simulink model "cc_architecture_model"  (R2024a)
settings: Solver=VariableStepAuto  StartTime=0.0  StopTime=10.0  RelTol=1e-3
settings Model: Creator=nevil  LastModifiedBy=nevil

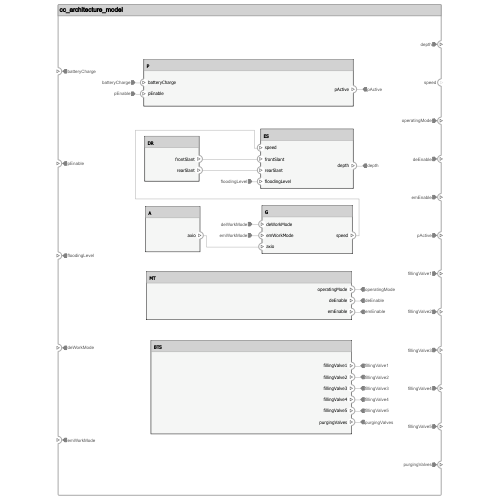
[thumbnail: Simulink's stored preview of the top-level diagram]
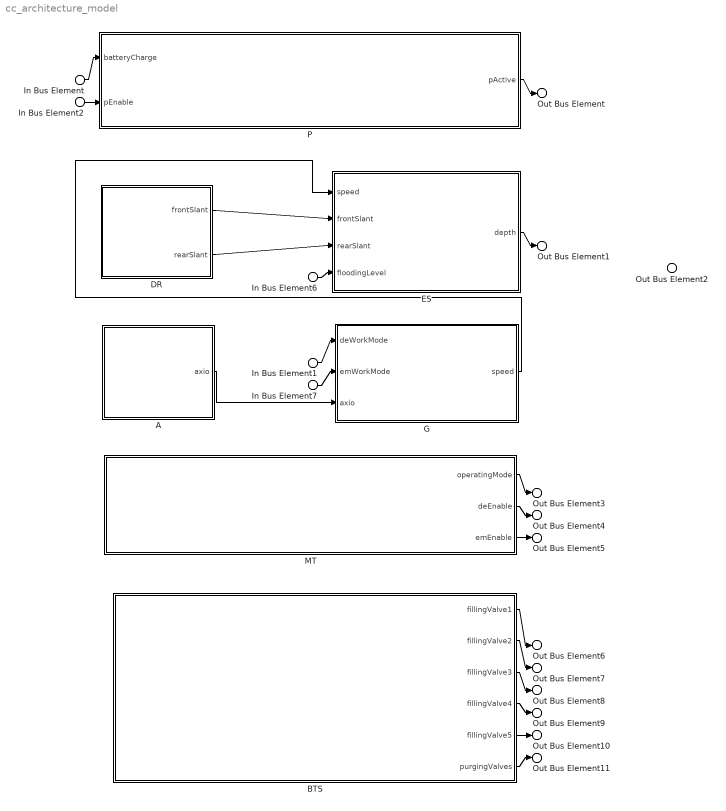
== system cc_architecture_model ==
  In Bus Element : Inport  PortName=batteryCharge
  In Bus Element2 : Inport  Port=2  PortName=pEnable
  In Bus Element6 : Inport  Port=3  PortName=floodingLevel
  In Bus Element1 : Inport  Port=4  PortName=deWorkMode
  In Bus Element7 : Inport  Port=5  PortName=emWorkMode
  A : Subsystem
      settings: PortSchema="{\"entries\":[{\"content\":{\"headerSize\":26,\"margin\":15,\"minimumSpacing\":25,\"sides\":[{\"content\":{},\"type\":\"ConnectorPlacement.EquallySpacedRectSide\",\"uuid\":\"55c3a500-c9db-403b-90f2-8c12a75bb2a5\"},{\"content\":{\"connectorIds\":[\"Out1\"],\"side\":\"RIGHT\"},\"type\":\"ConnectorPlacement.EquallySpacedRectSide\",\"uuid\":\"33fbbcf8-5fdb-46c8-86f1-27d61e7d7260\"},{\"content\":{\"side\":\"TOP\"},\"type\":\"ConnectorPlacement.EquallySpacedRectSide\",\"uuid\":\"56e8613f-dab0-46ca-a6c8-0c9dbbf33330\"}]},\"type\":\"ConnectorPlacement.EquallySpacedConnector\",\"uuid\":\"0944f535-9dc7-49a2-b8a9-c4d14048f3f3\"}],\"packageUris\":[\"http://schema.mathworks.com/mf0/Connector/R2020b\"],\"version\":\"1.0\"}"
  BTS : Subsystem
      settings: PortSchema="{\"entries\":[{\"content\":{\"headerSize\":26,\"margin\":15,\"minimumSpacing\":25,\"sides\":[{\"content\":{},\"type\":\"ConnectorPlacement.EquallySpacedRectSide\",\"uuid\":\"55c3a500-c9db-403b-90f2-8c12a75bb2a5\"},{\"content\":{\"connectorIds\":[\"Out1\",\"Out4\",\"Out3\",\"Out5\",\"Out2\",\"Out6\"],\"side\":\"RIGHT\"},\"type\":\"ConnectorPlacement.EquallySpacedRectSide\",\"uuid\":\"33fbbcf8-5fdb-46c8-86f1-27d61e7d7260\"},{\"content\":{\"side\":\"TOP\"},\"type\":\"ConnectorPlacement.EquallySpacedRectSide\",\"uuid\":\"56e8613f-dab0-46ca-a6c8-0c9dbbf33330\"}]},\"type\":\"ConnectorPlacement.EquallySpacedConnector\",\"uuid\":\"0944f535-9dc7-49a2-b8a9-c4d14048f3f3\"}],\"packageUris\":[\"http://schema.mathworks.com/mf0/Connector/R2020b\"],\"version\":\"1.0\"}"
  DR : Subsystem
      settings: PortSchema="{\"entries\":[{\"content\":{\"headerSize\":26,\"margin\":15,\"minimumSpacing\":25,\"sides\":[{\"content\":{},\"type\":\"ConnectorPlacement.EquallySpacedRectSide\",\"uuid\":\"55c3a500-c9db-403b-90f2-8c12a75bb2a5\"},{\"content\":{\"connectorIds\":[\"Out1\",\"Out2\"],\"side\":\"RIGHT\"},\"type\":\"ConnectorPlacement.EquallySpacedRectSide\",\"uuid\":\"33fbbcf8-5fdb-46c8-86f1-27d61e7d7260\"},{\"content\":{\"side\":\"TOP\"},\"type\":\"ConnectorPlacement.EquallySpacedRectSide\",\"uuid\":\"56e8613f-dab0-46ca-a6c8-0c9dbbf33330\"}]},\"type\":\"ConnectorPlacement.EquallySpacedConnector\",\"uuid\":\"0944f535-9dc7-49a2-b8a9-c4d14048f3f3\"}],\"packageUris\":[\"http://schema.mathworks.com/mf0/Connector/R2020b\"],\"version\":\"1.0\"}"
  ES : Subsystem
      settings: PortSchema="{\"entries\":[{\"content\":{\"headerSize\":26,\"margin\":15,\"minimumSpacing\":25,\"sides\":[{\"content\":{\"connectorIds\":[\"In1\",\"In2\",\"In3\",\"In4\"]},\"type\":\"ConnectorPlacement.EquallySpacedRectSide\",\"uuid\":\"fa34cfae-5758-447a-bbf8-61d94a7fad4b\"},{\"content\":{\"connectorIds\":[\"Out1\"],\"side\":\"RIGHT\"},\"type\":\"ConnectorPlacement.EquallySpacedRectSide\",\"uuid\":\"7d4a19cd-78f9-4f0a-b8b3-33613e9a47ea\"},{\"content\":{\"side\":\"TOP\"},\"type\":\"ConnectorPlacement.EquallySpacedRectSide\",\"uuid\":\"1bc8434e-3997-4d7a-991c-af8f97ade000\"}]},\"type\":\"ConnectorPlacement.EquallySpacedConnector\",\"uuid\":\"92e50b70-b613-4fba-b77c-cfd755548065\"}],\"packageUris\":[\"http://schema.mathworks.com/mf0/Connector/R2020b\"],\"version\":\"1.0\"}"
  G : Subsystem
      settings: PortSchema="{\"entries\":[{\"content\":{\"headerSize\":26,\"margin\":15,\"minimumSpacing\":25,\"sides\":[{\"content\":{\"connectorIds\":[\"In1\",\"In2\",\"In3\"]},\"type\":\"ConnectorPlacement.EquallySpacedRectSide\",\"uuid\":\"55c3a500-c9db-403b-90f2-8c12a75bb2a5\"},{\"content\":{\"connectorIds\":[\"Out1\"],\"side\":\"RIGHT\"},\"type\":\"ConnectorPlacement.EquallySpacedRectSide\",\"uuid\":\"33fbbcf8-5fdb-46c8-86f1-27d61e7d7260\"},{\"content\":{\"side\":\"TOP\"},\"type\":\"ConnectorPlacement.EquallySpacedRectSide\",\"uuid\":\"56e8613f-dab0-46ca-a6c8-0c9dbbf33330\"}]},\"type\":\"ConnectorPlacement.EquallySpacedConnector\",\"uuid\":\"0944f535-9dc7-49a2-b8a9-c4d14048f3f3\"}],\"packageUris\":[\"http://schema.mathworks.com/mf0/Connector/R2020b\"],\"version\":\"1.0\"}"
  MT : Subsystem
      settings: PortSchema="{\"entries\":[{\"content\":{\"headerSize\":26,\"margin\":15,\"minimumSpacing\":25,\"sides\":[{\"content\":{},\"type\":\"ConnectorPlacement.EquallySpacedRectSide\",\"uuid\":\"55c3a500-c9db-403b-90f2-8c12a75bb2a5\"},{\"content\":{\"connectorIds\":[\"Out1\",\"Out2\",\"Out3\"],\"side\":\"RIGHT\"},\"type\":\"ConnectorPlacement.EquallySpacedRectSide\",\"uuid\":\"33fbbcf8-5fdb-46c8-86f1-27d61e7d7260\"},{\"content\":{\"side\":\"TOP\"},\"type\":\"ConnectorPlacement.EquallySpacedRectSide\",\"uuid\":\"56e8613f-dab0-46ca-a6c8-0c9dbbf33330\"}]},\"type\":\"ConnectorPlacement.EquallySpacedConnector\",\"uuid\":\"0944f535-9dc7-49a2-b8a9-c4d14048f3f3\"}],\"packageUris\":[\"http://schema.mathworks.com/mf0/Connector/R2020b\"],\"version\":\"1.0\"}"
  P : Subsystem
      settings: PortSchema="{\"entries\":[{\"content\":{\"headerSize\":26,\"margin\":15,\"minimumSpacing\":25,\"sides\":[{\"content\":{\"connectorIds\":[\"In1\",\"In2\"]},\"type\":\"ConnectorPlacement.EquallySpacedRectSide\",\"uuid\":\"fa34cfae-5758-447a-bbf8-61d94a7fad4b\"},{\"content\":{\"connectorIds\":[\"Out1\"],\"side\":\"RIGHT\"},\"type\":\"ConnectorPlacement.EquallySpacedRectSide\",\"uuid\":\"7d4a19cd-78f9-4f0a-b8b3-33613e9a47ea\"},{\"content\":{\"side\":\"TOP\"},\"type\":\"ConnectorPlacement.EquallySpacedRectSide\",\"uuid\":\"1bc8434e-3997-4d7a-991c-af8f97ade000\"}]},\"type\":\"ConnectorPlacement.EquallySpacedConnector\",\"uuid\":\"92e50b70-b613-4fba-b77c-cfd755548065\"}],\"packageUris\":[\"http://schema.mathworks.com/mf0/Connector/R2020b\"],\"version\":\"1.0\"}"
  Out Bus Element1 : Outport  PortName=depth
  Out Bus Element2 : Outport  Port=2  PortName=speed
  Out Bus Element3 : Outport  Port=3  PortName=operatingMode
  Out Bus Element4 : Outport  Port=4  PortName=deEnable
  Out Bus Element5 : Outport  Port=5  PortName=emEnable
  Out Bus Element : Outport  Port=6  PortName=pActive
  Out Bus Element6 : Outport  Port=7  PortName=fillingValve1
  Out Bus Element7 : Outport  Port=8  PortName=fillingValve2
  Out Bus Element8 : Outport  Port=9  PortName=fillingValve3
  Out Bus Element9 : Outport  Port=10  PortName=fillingValve4
  Out Bus Element10 : Outport  Port=11  PortName=fillingValve5
  Out Bus Element11 : Outport  Port=12  PortName=purgingValves
  wires:
  A/1(axio) -> G/3(axio)
  In Bus Element/1 -> P/1(batteryCharge)
  In Bus Element2/1 -> P/2(pEnable)
  In Bus Element6/1 -> ES/4(floodingLevel)
  In Bus Element1/1 -> G/1(deWorkMode)
  In Bus Element7/1 -> G/2(emWorkMode)
  P/1(pActive) -> Out Bus Element/1
  ES/1(depth) -> Out Bus Element1/1
  G/1(speed) -> ES/1(speed)
  DR/1(frontSlant) -> ES/2(frontSlant)
  DR/2(rearSlant) -> ES/3(rearSlant)
  MT/2(deEnable) -> Out Bus Element4/1
  MT/3(emEnable) -> Out Bus Element5/1
  MT/1(operatingMode) -> Out Bus Element3/1
  BTS/1(fillingValve1) -> Out Bus Element6/1
  BTS/4(fillingValve2) -> Out Bus Element7/1
  BTS/3(fillingValve3) -> Out Bus Element8/1
  BTS/5(fillingValve4) -> Out Bus Element9/1
  BTS/2(fillingValve5) -> Out Bus Element10/1
  BTS/6(purgingValves) -> Out Bus Element11/1

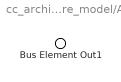
== system cc_architecture_model/A ==
  Bus Element Out1 : Outport  PortName=axio

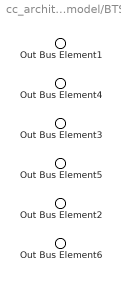
== system cc_architecture_model/BTS ==
  Out Bus Element1 : Outport  PortName=fillingValve1
  Out Bus Element2 : Outport  Port=2  PortName=fillingValve5
  Out Bus Element3 : Outport  Port=3  PortName=fillingValve3
  Out Bus Element4 : Outport  Port=4  PortName=fillingValve2
  Out Bus Element5 : Outport  Port=5  PortName=fillingValve4
  Out Bus Element6 : Outport  Port=6  PortName=purgingValves

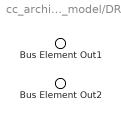
== system cc_architecture_model/DR ==
  Bus Element Out1 : Outport  PortName=frontSlant
  Bus Element Out2 : Outport  Port=2  PortName=rearSlant

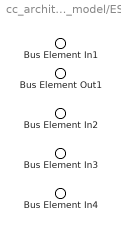
== system cc_architecture_model/ES ==
  Bus Element In1 : Inport  PortName=speed
  Bus Element In2 : Inport  Port=2  PortName=frontSlant
  Bus Element In3 : Inport  Port=3  PortName=rearSlant
  Bus Element In4 : Inport  Port=4  PortName=floodingLevel
  Bus Element Out1 : Outport  PortName=depth

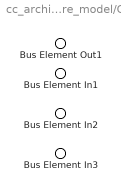
== system cc_architecture_model/G ==
  Bus Element In1 : Inport  PortName=deWorkMode
  Bus Element In2 : Inport  Port=2  PortName=emWorkMode
  Bus Element In3 : Inport  Port=3  PortName=axio
  Bus Element Out1 : Outport  PortName=speed

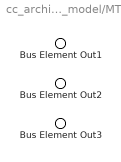
== system cc_architecture_model/MT ==
  Bus Element Out1 : Outport  PortName=operatingMode
  Bus Element Out2 : Outport  Port=2  PortName=deEnable
  Bus Element Out3 : Outport  Port=3  PortName=emEnable

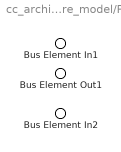
== system cc_architecture_model/P ==
  Bus Element In1 : Inport  PortName=batteryCharge
  Bus Element In2 : Inport  Port=2  PortName=pEnable
  Bus Element Out1 : Outport  PortName=pActive
